simulink model "aero_dap3dof"  (Simulink 6.0)
settings: Solver=ode45  SolverMode=SingleTasking  StartTime=0  StopTime=25  FixedStep=clockt/4  RelTol=1e-3  AbsTol=1e-6
PreLoadFcn:
  | aero_dap3dofdata
values from neighbouring files (symbols this model uses):
  DB = u(6)    [aero_phaseplane.m]
  delt = 0.1    [aero_pointer_tracker.m]
  I = find(diff(Mode.signals.values)~=0)    [aero_guid_plot.m]
undefined symbols (not defined in the file or in its folder): alph1, alphs1, alphsu, alphsv, alphu, alphv, Force, L_arm, tmin
libraries: simulink x2
Description:
  | This model was featured in "Fly Me to the Moon - Then and Now", the story of the digital autopilot in the Lunar Module from the Summer 1999 issue of "MATLAB News & Notes".  You can read the article at:
  | 
  |  http://www.mathworks.com/company/newsletter/news_notes/sum99/lunar_module.html
CloseFcn:
  | h=findobj('type','figure','Name','aero_dap3dof');if ~isempty(h);close(h);end
settings Model: RequirementInfo=9  CovMetricSettings=d  Creator=The MathWorks Inc.  LastModifiedBy=batserve  ExtModeTrigMode=oneshot  ExtModeArmWhenConnect=off  ExtModeAutoUpdateStatusClock=off  ProdHWDeviceType=Specified
settings DataIOCC: LimitDataPoints=off  SignalLoggingName=logsOut
settings OptimizationCC: BlockReduction=off  BooleanDataType=off
settings DebuggingCC: CheckExecutionContextPreStartOutputMsg=on  CheckExecutionContextRuntimeOutputMsg=on  SolverPrmCheckMsg=none
settings HardwareCC: ProdHWDeviceType=Specified
settings RTWCC: TemplateMakefile=grt_vc.tmf

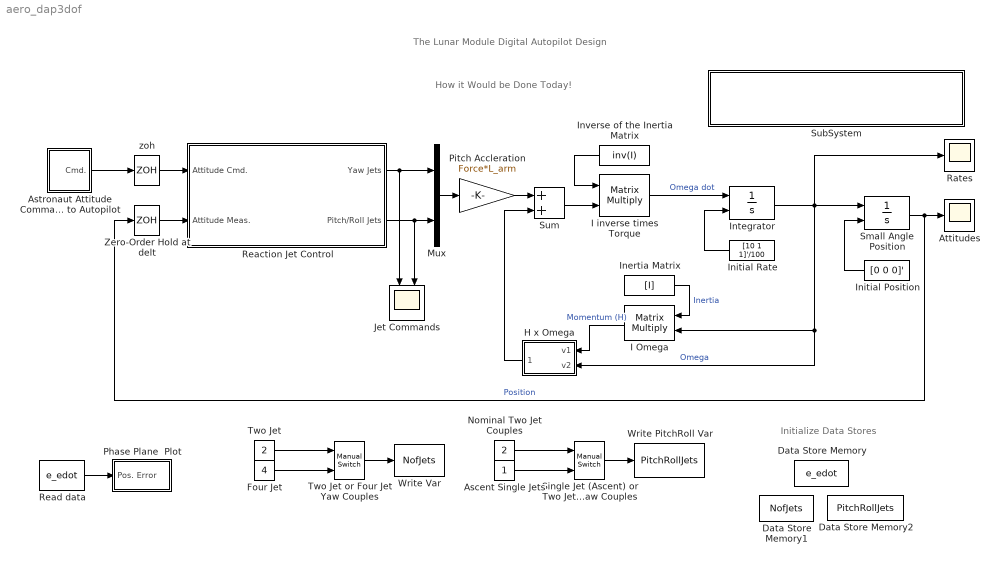
== system aero_dap3dof ==
  note: The Lunar Module Digital Autopilot Design
  note: How it Would be Done Today!
  note: Initialize Data Stores
  Ascent Single Jets : Constant
  Astronaut Attitude Command to Autopilot : Subsystem  PropExecContextAcrossSSBoundary=on
  Attitudes : Scope
      settings: YMin=0  YMax=0.12
  Data Store Memory : DataStoreMemory  DialogController=Simulink.DDGSource  DataStoreName=e_edot  InitialValue=[0 0]
  Data Store Memory1 : DataStoreMemory  DialogController=Simulink.DDGSource  DataStoreName=NofJets  InitialValue=2
  Data Store Memory2 : DataStoreMemory  DialogController=Simulink.DDGSource  DataStoreName=PitchRollJets  InitialValue=2
  Four Jet : Constant  Value=4
  H x Omega : Subsystem  Orientation=left  PropExecContextAcrossSSBoundary=on
      mask Type: Vector Cross Product
      mask Description: This block computes the vector cross product of the first input with the second input.  The output is then z= v1 x v2.
  I Omega : Product  Orientation=left  Multiplication=Matrix(*)  SaturateOnIntegerOverflow=on  RndMeth=Zero  InputSameDT=on
  I inverse times Torque : Product  Multiplication=Matrix(*)  SaturateOnIntegerOverflow=on  RndMeth=Zero  InputSameDT=on
  Inertia Matrix : Constant  Value=[I]  VectorParams1D=off
  Initial Position : Constant  Orientation=left  Value=[0 0 0]'  VectorParams1D=off
  Initial Rate : Constant  Orientation=left  Value=[10 1 1]'/100  VectorParams1D=off
  Integrator : Integrator  InitialConditionSource=external
  Inverse of the Inertia Matrix : Constant  Orientation=left  Value=inv(I)  VectorParams1D=off
  Jet Commands : Scope  NumInputPorts=2
      settings: Orientation=down  TickLabels=on  TimeRange=9.999999999999998  YMin=-3~-3  YMax=3~3  DataFormat=Array  MaxDataPoints=10000
  Mux : Mux  Inputs=2
  Nominal Two Jet Couples : Constant  Value=2
  Phase Plane  Plot : Subsystem  PropExecContextAcrossSSBoundary=on
  Pitch Accleration : Gain  Gain=Force*L_arm  SaturateOnIntegerOverflow=on
  Rates : Scope
      settings: YMin=-0.075  YMax=0.125
  Reaction Jet Control : Subsystem  AncestorBlock=librcs/Reaction Jet Control  PropExecContextAcrossSSBoundary=on
  Read data : DataStoreRead  DialogController=Simulink.DDGSource  DataStoreName=e_edot  SampleTime=delt
  Single Jet (Ascent) or Two Jet Yaw Couples : simulink/Signal Routing/Manual Switch  sw=1  action=0
  Small Angle Position : Integrator  InitialConditionSource=external
  SubSystem : Subsystem  PropExecContextAcrossSSBoundary=on
      mask init:
      | dispstr = sprintf('Read the "News & Notes" article\nabout this model over the web.\n(Double-Click Here)');
      settings: OpenFcn=web http://www.mathworks.com/company/newsletter/news_notes/sum99/lunar_module.html
      mask Display: disp(dispstr)
  Sum : Sum  SaturateOnIntegerOverflow=on  InputSameDT=on
  Two Jet : Constant  Value=2
  Two Jet or Four Jet Yaw Couples : simulink/Signal Routing/Manual Switch  sw=1  action=0
  Write PitchRoll Var : DataStoreWrite  DialogController=Simulink.DDGSource  DataStoreName=PitchRollJets  SampleTime=-1
  Write Var : DataStoreWrite  DialogController=Simulink.DDGSource  DataStoreName=NofJets  SampleTime=-1
  Zero-Order Hold at delt : ZeroOrderHold  SampleTime=delt
  zoh : ZeroOrderHold  SampleTime=delt
  wires:
  Inverse of the Inertia Matrix/1 -> I inverse times Torque/1
  I inverse times Torque/1 -> Integrator/1  "Omega dot"
  Inertia Matrix/1 -> I Omega/1  "Inertia"
  Initial Rate/1 -> Integrator/2
  Initial Position/1 -> Small Angle Position/2
  Integrator/1 -> Small Angle Position/1, I Omega/2, H x Omega/2(v2), Rates/1  "Omega"
  Small Angle Position/1 -> Attitudes/1, Zero-Order Hold at delt/1  "Position"
  Sum/1 -> I inverse times Torque/2
  I Omega/1 -> H x Omega/1(v1)  "Momentum (H)"
  H x Omega/1(v1 x v2) -> Sum/2
  Astronaut Attitude Command to Autopilot/1(Cmd.) -> zoh/1
  Pitch Accleration/1 -> Sum/1
  Mux/1 -> Pitch Accleration/1
  Reaction Jet Control/1(Yaw Jets) -> Mux/1, Jet Commands/1
  Reaction Jet Control/2(Pitch/Roll Jets) -> Mux/2, Jet Commands/2
  zoh/1 -> Reaction Jet Control/1(Attitude Cmd.)
  Zero-Order Hold at delt/1 -> Reaction Jet Control/2(Attitude Meas.)
  Ascent Single Jets/1 -> Single Jet (Ascent) or Two Jet Yaw Couples/2
  Nominal Two Jet Couples/1 -> Single Jet (Ascent) or Two Jet Yaw Couples/1
  Single Jet (Ascent) or Two Jet Yaw Couples/1 -> Write PitchRoll Var/1
  Four Jet/1 -> Two Jet or Four Jet Yaw Couples/2
  Two Jet/1 -> Two Jet or Four Jet Yaw Couples/1
  Two Jet or Four Jet Yaw Couples/1 -> Write Var/1
  Read data/1 -> Phase Plane  Plot/1(Pos. Error)

== system aero_dap3dof/Astronaut Attitude Command to Autopilot ==
  Attitude Cmd at t=0 : Constant  Value=[0 0 0]'  VectorParams1D=off
  Attitude Cmd at t=step : Constant  Value=[0.03 0.05 0.1]'  VectorParams1D=off
  Step : Step  Time=0.25  SampleTime=0
  Switch : Switch  Threshold=0.5  SaturateOnIntegerOverflow=on  InputSameDT=on
  Cmd. : Outport
  wires:
  Step/1 -> Switch/2
  Attitude Cmd at t=step/1 -> Switch/1
  Attitude Cmd at t=0/1 -> Switch/3
  Switch/1 -> Cmd./1

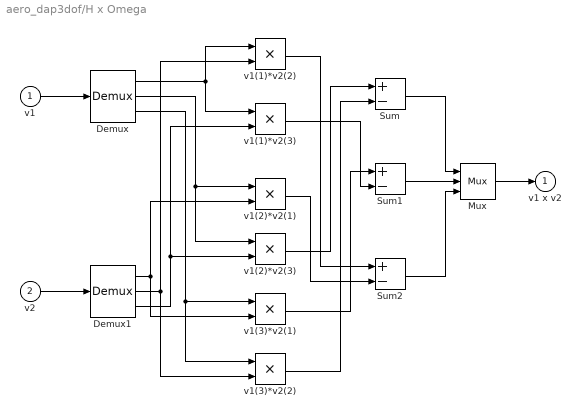
== system aero_dap3dof/H x Omega ==
  v1 : Inport  Port=1  LatchInput=off
  v2 : Inport  Port=2  LatchInput=off
  Demux : Demux  Outputs=3
  Demux1 : Demux  Outputs=3
  Mux : Mux  Inputs=3
  Sum : Sum  Inputs=+-  SaturateOnIntegerOverflow=on  InputSameDT=on
  Sum1 : Sum  Inputs=+-  SaturateOnIntegerOverflow=on  InputSameDT=on
  Sum2 : Sum  Inputs=+-  SaturateOnIntegerOverflow=on  InputSameDT=on
  v1(1)*v2(2) : Product  SaturateOnIntegerOverflow=on  RndMeth=Zero  InputSameDT=on
  v1(1)*v2(3) : Product  SaturateOnIntegerOverflow=on  RndMeth=Zero  InputSameDT=on
  v1(2)*v2(1) : Product  SaturateOnIntegerOverflow=on  RndMeth=Zero  InputSameDT=on
  v1(2)*v2(3) : Product  SaturateOnIntegerOverflow=on  RndMeth=Zero  InputSameDT=on
  v1(3)*v2(1) : Product  SaturateOnIntegerOverflow=on  RndMeth=Zero  InputSameDT=on
  v1(3)*v2(2) : Product  SaturateOnIntegerOverflow=on  RndMeth=Zero  InputSameDT=on
  v1 x v2 : Outport  InitialOutput=0
  wires:
  v1/1 -> Demux/1
  Demux/3 -> v1(3)*v2(1)/1, v1(3)*v2(2)/1
  v2/1 -> Demux1/1
  Demux1/1 -> v1(2)*v2(1)/2, v1(3)*v2(1)/2
  Demux1/2 -> v1(3)*v2(2)/2, v1(1)*v2(2)/2
  Demux1/3 -> v1(2)*v2(3)/2, v1(1)*v2(3)/2
  Demux/1 -> v1(1)*v2(2)/1, v1(1)*v2(3)/1
  Demux/2 -> v1(2)*v2(1)/1, v1(2)*v2(3)/1
  Mux/1 -> v1 x v2/1
  Sum/1 -> Mux/1
  Sum1/1 -> Mux/2
  Sum2/1 -> Mux/3
  v1(2)*v2(3)/1 -> Sum/1
  v1(3)*v2(2)/1 -> Sum/2
  v1(3)*v2(1)/1 -> Sum1/1
  v1(1)*v2(3)/1 -> Sum1/2
  v1(1)*v2(2)/1 -> Sum2/1
  v1(2)*v2(1)/1 -> Sum2/2

== system aero_dap3dof/Phase Plane  Plot ==
  Pos. Error : Inport  Port=1  LatchInput=off
  Constant : Constant  Value=alph1
  Constant1 : Constant  Value=alphs1
  Constants for Plot : Constant  Value=DB
  Digital Clock : DigitalClock  SampleTime=delt
  MATLAB Fcn : MATLABFcn  MATLABFcn=aero_phaseplane  OutputDimensions=0
  Mux1 : Mux  Inputs=5
  wires:
  Mux1/1 -> MATLAB Fcn/1
  Pos. Error/1 -> Mux1/1
  Digital Clock/1 -> Mux1/2
  Constants for Plot/1 -> Mux1/5
  Constant/1 -> Mux1/3
  Constant1/1 -> Mux1/4

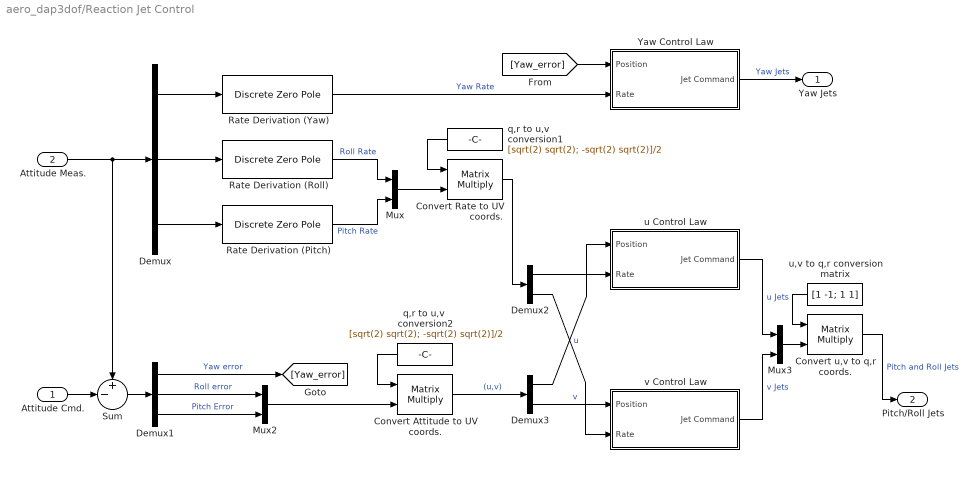
== system aero_dap3dof/Reaction Jet Control ==
  Attitude Cmd. : Inport  Port=1  LatchInput=off
  Attitude Meas. : Inport  Port=2  LatchInput=off
  Convert Attitude to UV coords. : Product  Multiplication=Matrix(*)  SaturateOnIntegerOverflow=on  RndMeth=Zero  InputSameDT=on
  Convert Rate to UV coords. : Product  Multiplication=Matrix(*)  SaturateOnIntegerOverflow=on  RndMeth=Zero  InputSameDT=on
  Convert u,v to q,r coords. : Product  Multiplication=Matrix(*)  SaturateOnIntegerOverflow=on  RndMeth=Zero  InputSameDT=on
  Demux : Demux  Outputs=3
  Demux1 : Demux  Outputs=3
  Demux2 : Demux  Outputs=2
  Demux3 : Demux  Outputs=2
  Mux : Mux  Inputs=2
  Mux2 : Mux  Inputs=2
  Mux3 : Mux  Inputs=2
  Rate Derivation (Pitch) : DiscreteZeroPole  Poles=[0]  Gain=1/delt  SampleTime=-1
  Rate Derivation (Roll) : DiscreteZeroPole  Poles=[0]  Gain=1/delt  SampleTime=-1
  Rate Derivation (Yaw) : DiscreteZeroPole  Poles=[0]  Gain=1/delt  SampleTime=-1
  Sum : Sum  Inputs=+-|  SaturateOnIntegerOverflow=on  InputSameDT=on
  Yaw Control Law : Subsystem  AncestorBlock=libdap/Yaw Control Law  PropExecContextAcrossSSBoundary=on  mask(Control Law){alph=alph1, alphs=alphs1, DB=DB, tmin=tmin, delt=delt}
      mask prompts: alph "Single Jet Accel:"; alphs "Single Jet Switch Curve Accel:"; DB "Dead Band:"; tmin "Min Jet On Time:"; delt "Sample Time:"
      mask help: Implements Control Law for the LM. Works for yaw, u and v jet axes.
  q,r to u,v  conversion1 : Constant  Orientation=left  Value=[sqrt(2) sqrt(2); -sqrt(2) sqrt(2)]/2  VectorParams1D=off
  q,r to u,v  conversion2 : Constant  Orientation=left  Value=[sqrt(2) sqrt(2); -sqrt(2) sqrt(2)]/2  VectorParams1D=off
  u Control Law : Subsystem  AncestorBlock=libdap/Pitch Roll Control Law  PropExecContextAcrossSSBoundary=on  mask(Control Law){alph=alphu, alphs=alphsu, DB=DB, tmin=tmin, delt=delt}
      mask prompts: alph "Single Jet Accel:"; alphs "Single Jet Switch Curve Accel:"; DB "Dead Band:"; tmin "Min. Jet On Time:"; delt "Sample Time:"
      mask help: Implements Control Law for the LM. Works for yaw, u and v jet axes.
  u,v to q,r conversion matrix : Constant  Orientation=left  Value=[1 -1; 1 1]  VectorParams1D=off
  v Control Law : Subsystem  AncestorBlock=libdap/Pitch Roll Control Law  PropExecContextAcrossSSBoundary=on  mask(Control Law){alph=alphv, alphs=alphsv, DB=DB, tmin=tmin, delt=delt}
      mask prompts: alph "Single Jet Accel:"; alphs "Single Jet Switch Curve Accel:"; DB "Dead Band:"; tmin "Min. Jet On Time:"; delt "Sample Time:"
      mask help: Implements Control Law for the LM. Works for yaw, u and v jet axes.
  Yaw Jets : Outport  InitialOutput=0
  Pitch/Roll Jets : Outport  Port=2  InitialOutput=0
  wires:
  q,r to u,v  conversion2/1 -> Convert Attitude to UV coords./1
  q,r to u,v  conversion1/1 -> Convert Rate to UV coords./1
  Rate Derivation (Pitch)/1 -> Mux/2  "Pitch Rate"
  Rate Derivation (Roll)/1 -> Mux/1  "Roll Rate"
  Demux/2 -> Rate Derivation (Roll)/1
  Demux/3 -> Rate Derivation (Pitch)/1
  Demux/1 -> Rate Derivation (Yaw)/1
  Mux/1 -> Convert Rate to UV coords./2
  Attitude Meas./1 -> Demux/1, Sum/1
  Rate Derivation (Yaw)/1 -> Yaw Control Law/2(Rate)  "Yaw Rate"
  Yaw Control Law/1(Jet Command) -> Yaw Jets/1  "Yaw Jets"
  [Yaw_error] -> Yaw Control Law/1(Position)
  Sum/1 -> Demux1/1
  Demux1/2 -> Mux2/1  "Roll error"
  Demux1/3 -> Mux2/2  "Pitch Error"
  Convert Rate to UV coords./1 -> Demux2/1
  Convert Attitude to UV coords./1 -> Demux3/1  "(u,v)"
  Mux2/1 -> Convert Attitude to UV coords./2
  Attitude Cmd./1 -> Sum/2
  v Control Law/1(Jet Command) -> Mux3/2  "v Jets"
  u Control Law/1(Jet Command) -> Mux3/1  "u Jets"
  Demux3/2 -> v Control Law/1(Position)  "v"
  Demux2/1 -> u Control Law/2(Rate)
  Demux1/1 -> [Yaw_error]  "Yaw error"
  Demux2/2 -> v Control Law/2(Rate)
  Mux3/1 -> Convert u,v to q,r coords./2
  u,v to q,r conversion matrix/1 -> Convert u,v to q,r coords./1
  Convert u,v to q,r coords./1 -> Pitch/Roll Jets/1  "Pitch and Roll Jets"
  Demux3/1 -> u Control Law/1(Position)  "u"

== system aero_dap3dof/SubSystem ==

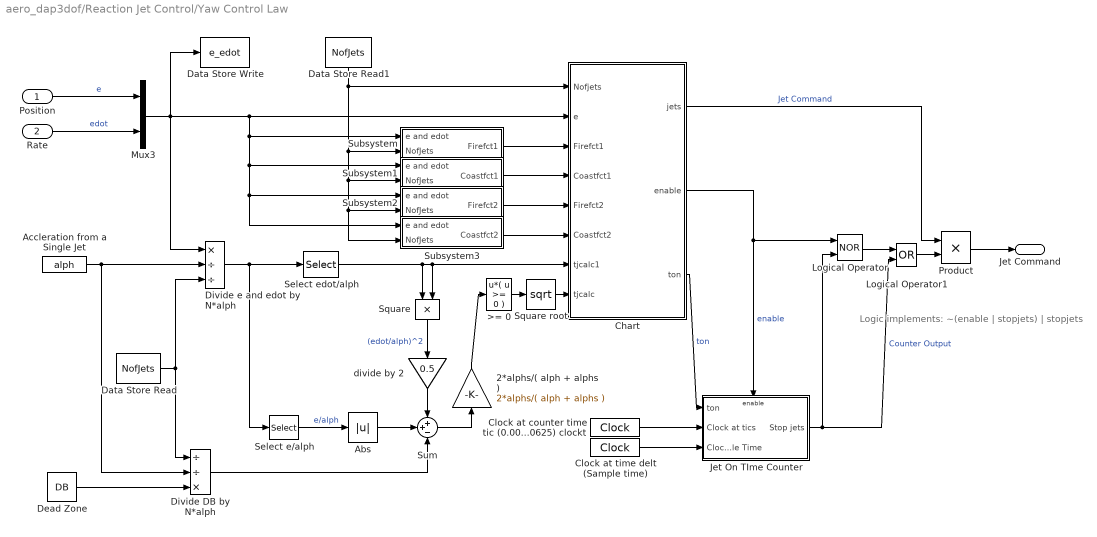
== system aero_dap3dof/Reaction Jet Control/Yaw Control Law ==
  note: Logic implements:
      | ~(enable | stopjets) | stopjets
  Position : Inport  Port=1  LatchInput=off
  Rate : Inport  Port=2  LatchInput=off
  2*alphs/( alph + alphs ) : Gain  Orientation=up  Gain=2*alphs/( alph + alphs )  SaturateOnIntegerOverflow=on
  >= 0 : Fcn  Expr=u*( u >= 0 )
  Abs : Abs  SaturateOnIntegerOverflow=on
  Accleration from a Single Jet : Constant  Value=alph
  Chart : Stateflow chart  PropExecContextAcrossSSBoundary=on
  Clock at counter time tic (0.000625) clockt : DigitalClock  SampleTime=0.000625
  Clock at time delt (Sample time) : DigitalClock  SampleTime=delt
  Data Store Read : DataStoreRead  DialogController=Simulink.DDGSource  DataStoreName=NofJets  SampleTime=delt
  Data Store Read1 : DataStoreRead  Orientation=down  DialogController=Simulink.DDGSource  DataStoreName=NofJets  SampleTime=delt
  Data Store Write : DataStoreWrite  DialogController=Simulink.DDGSource  DataStoreName=e_edot  SampleTime=-1
  Dead Zone : Constant  Value=DB
  Divide e and edot by N*alph : Product  Inputs=*//  SaturateOnIntegerOverflow=on  RndMeth=Zero  InputSameDT=on
  Divide DB by N*alph : Product  Inputs=//*  SaturateOnIntegerOverflow=on  RndMeth=Zero  InputSameDT=on
  Jet On TIme Counter : Subsystem  TreatAsAtomicUnit=on  PropExecContextAcrossSSBoundary=on
  Logical Operator : Logic  Operator=NOR
  Logical Operator1 : Logic  Operator=OR
  Mux3 : Mux  Inputs=2
  Product : Product  SaturateOnIntegerOverflow=on  RndMeth=Zero  InputSameDT=on
  Select e/alph : Selector  Elements=[1]  InputPortWidth=2
  Select edot/alph : Selector  Elements=[2]  InputPortWidth=2
  Square : Product  Orientation=down  SaturateOnIntegerOverflow=on  RndMeth=Zero  InputSameDT=on
  Square root : Math  Operator=sqrt  SaturateOnIntegerOverflow=on
  Subsystem : Subsystem  PropExecContextAcrossSSBoundary=on
  Subsystem1 : Subsystem  PropExecContextAcrossSSBoundary=on
  Subsystem2 : Subsystem  PropExecContextAcrossSSBoundary=on
  Subsystem3 : Subsystem  PropExecContextAcrossSSBoundary=on
  Sum : Sum  Inputs=++-  SaturateOnIntegerOverflow=on  InputSameDT=on
  divide by 2 : Gain  Orientation=down  Gain=0.5  SaturateOnIntegerOverflow=on
  Jet Command : Outport  InitialOutput=0
  wires:
  >= 0/1 -> Square root/1
  2*alphs/( alph + alphs )/1 -> >= 0/1
  Data Store Read1/1 -> Subsystem3/2(NofJets), Subsystem2/2(NofJets), Subsystem1/2(NofJets), Subsystem/2(NofJets), Chart/1(Nofjets)
  Rate/1 -> Mux3/2  "edot"
  Position/1 -> Mux3/1  "e"
  Mux3/1 -> Data Store Write/1, Chart/2(e), Divide e and edot by N*alph/1, Subsystem/1(e and edot), Subsystem1/1(e and edot), Subsystem2/1(e and edot), Subsystem3/1(e and edot)
  Square/1 -> divide by 2/1  "(edot/alph)^2"
  Square root/1 -> Chart/8(tjcalc)
  Chart/1(jets) -> Product/1  "Jet Command"
  Select edot/alph/1 -> Square/1, Chart/7(tjcalc1), Square/2
  Select e/alph/1 -> Abs/1  "e/alph"
  divide by 2/1 -> Sum/1
  Sum/1 -> 2*alphs/( alph + alphs )/1
  Abs/1 -> Sum/2
  Divide e and edot by N*alph/1 -> Select edot/alph/1, Select e/alph/1
  Data Store Read/1 -> Divide e and edot by N*alph/3, Divide DB by N*alph/1
  Accleration from a Single Jet/1 -> Divide e and edot by N*alph/2, Divide DB by N*alph/2
  Dead Zone/1 -> Divide DB by N*alph/3
  Divide DB by N*alph/1 -> Sum/3
  Chart/2(enable) -> Jet On TIme Counter/Enable, Logical Operator/1  "enable"
  Logical Operator1/1 -> Product/2
  Chart/3(ton) -> Jet On TIme Counter/1(ton)  "ton"
  Clock at counter time tic (0.000625) clockt/1 -> Jet On TIme Counter/2(Clock at tics)
  Clock at time delt (Sample time)/1 -> Jet On TIme Counter/3(Clock at Sample Time)
  Jet On TIme Counter/1(Stop jets) -> Logical Operator/2, Logical Operator1/2  "Counter Output"
  Logical Operator/1 -> Logical Operator1/1
  Subsystem3/1(Coastfct2) -> Chart/6(Coastfct2)
  Subsystem2/1(Firefct2) -> Chart/5(Firefct2)
  Subsystem1/1(Coastfct1) -> Chart/4(Coastfct1)
  Subsystem/1(Firefct1) -> Chart/3(Firefct1)
  Product/1 -> Jet Command/1

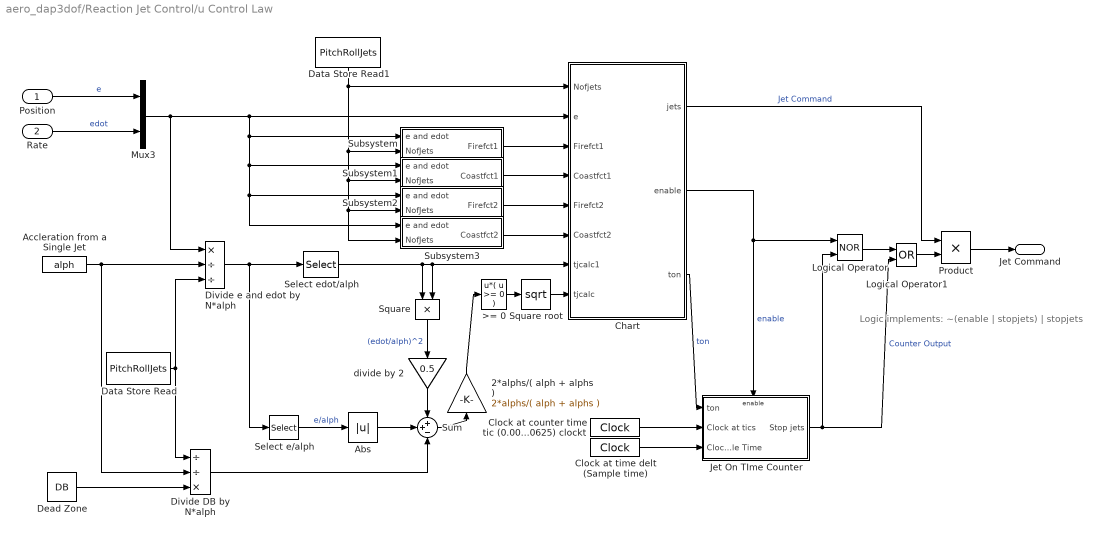
== system aero_dap3dof/Reaction Jet Control/u Control Law ==
  note: Logic implements:
      | ~(enable | stopjets) | stopjets
  Position : Inport  Port=1  LatchInput=off
  Rate : Inport  Port=2  LatchInput=off
  2*alphs/( alph + alphs ) : Gain  Orientation=up  Gain=2*alphs/( alph + alphs )  SaturateOnIntegerOverflow=on
  >= 0 : Fcn  Expr=u*( u >= 0 )
  Abs : Abs  SaturateOnIntegerOverflow=on
  Accleration from a Single Jet : Constant  Value=alph
  Chart : Stateflow chart  PropExecContextAcrossSSBoundary=on
  Clock at counter time tic (0.000625) clockt : DigitalClock  SampleTime=0.000625
  Clock at time delt (Sample time) : DigitalClock  SampleTime=delt
  Data Store Read : DataStoreRead  DialogController=Simulink.DDGSource  DataStoreName=PitchRollJets  SampleTime=delt
  Data Store Read1 : DataStoreRead  Orientation=down  DialogController=Simulink.DDGSource  DataStoreName=PitchRollJets  SampleTime=delt
  Dead Zone : Constant  Value=DB
  Divide e and edot by N*alph : Product  Inputs=*//  SaturateOnIntegerOverflow=on  RndMeth=Zero  InputSameDT=on
  Divide DB by N*alph : Product  Inputs=//*  SaturateOnIntegerOverflow=on  RndMeth=Zero  InputSameDT=on
  Jet On TIme Counter : Subsystem  TreatAsAtomicUnit=on  PropExecContextAcrossSSBoundary=on
  Logical Operator : Logic  Operator=NOR
  Logical Operator1 : Logic  Operator=OR
  Mux3 : Mux  Inputs=2
  Product : Product  SaturateOnIntegerOverflow=on  RndMeth=Zero  InputSameDT=on
  Select e/alph : Selector  Elements=[1]  InputPortWidth=2
  Select edot/alph : Selector  Elements=[2]  InputPortWidth=2
  Square : Product  Orientation=down  SaturateOnIntegerOverflow=on  RndMeth=Zero  InputSameDT=on
  Square root : Math  Operator=sqrt  SaturateOnIntegerOverflow=on
  Subsystem : Subsystem  PropExecContextAcrossSSBoundary=on
  Subsystem1 : Subsystem  PropExecContextAcrossSSBoundary=on
  Subsystem2 : Subsystem  PropExecContextAcrossSSBoundary=on
  Subsystem3 : Subsystem  PropExecContextAcrossSSBoundary=on
  Sum : Sum  Inputs=++-  SaturateOnIntegerOverflow=on  InputSameDT=on
  divide by 2 : Gain  Orientation=down  Gain=0.5  SaturateOnIntegerOverflow=on
  Jet Command : Outport  InitialOutput=0
  wires:
  >= 0/1 -> Square root/1
  2*alphs/( alph + alphs )/1 -> >= 0/1
  Product/1 -> Jet Command/1
  Subsystem/1(Firefct1) -> Chart/3(Firefct1)
  Subsystem1/1(Coastfct1) -> Chart/4(Coastfct1)
  Subsystem2/1(Firefct2) -> Chart/5(Firefct2)
  Subsystem3/1(Coastfct2) -> Chart/6(Coastfct2)
  Logical Operator/1 -> Logical Operator1/1
  Jet On TIme Counter/1(Stop jets) -> Logical Operator1/2, Logical Operator/2  "Counter Output"
  Clock at time delt (Sample time)/1 -> Jet On TIme Counter/3(Clock at Sample Time)
  Clock at counter time tic (0.000625) clockt/1 -> Jet On TIme Counter/2(Clock at tics)
  Chart/3(ton) -> Jet On TIme Counter/1(ton)  "ton"
  Logical Operator1/1 -> Product/2
  Chart/2(enable) -> Logical Operator/1, Jet On TIme Counter/Enable  "enable"
  Divide DB by N*alph/1 -> Sum/3
  Dead Zone/1 -> Divide DB by N*alph/3
  Accleration from a Single Jet/1 -> Divide DB by N*alph/2, Divide e and edot by N*alph/2
  Data Store Read/1 -> Divide DB by N*alph/1, Divide e and edot by N*alph/3
  Divide e and edot by N*alph/1 -> Select e/alph/1, Select edot/alph/1
  Abs/1 -> Sum/2
  Sum/1 -> 2*alphs/( alph + alphs )/1
  divide by 2/1 -> Sum/1
  Select e/alph/1 -> Abs/1  "e/alph"
  Select edot/alph/1 -> Square/2, Chart/7(tjcalc1), Square/1
  Chart/1(jets) -> Product/1  "Jet Command"
  Square root/1 -> Chart/8(tjcalc)
  Square/1 -> divide by 2/1  "(edot/alph)^2"
  Mux3/1 -> Subsystem3/1(e and edot), Subsystem2/1(e and edot), Subsystem1/1(e and edot), Subsystem/1(e and edot), Divide e and edot by N*alph/1, Chart/2(e)
  Position/1 -> Mux3/1  "e"
  Rate/1 -> Mux3/2  "edot"
  Data Store Read1/1 -> Chart/1(Nofjets), Subsystem/2(NofJets), Subsystem1/2(NofJets), Subsystem2/2(NofJets), Subsystem3/2(NofJets)

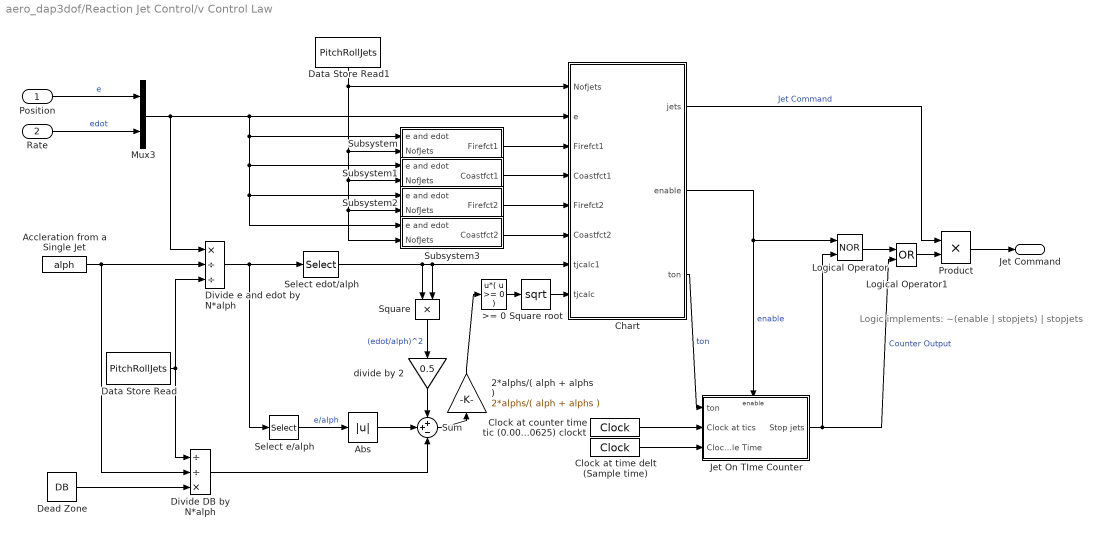
== system aero_dap3dof/Reaction Jet Control/v Control Law ==
  note: Logic implements:
      | ~(enable | stopjets) | stopjets
  Position : Inport  Port=1  LatchInput=off
  Rate : Inport  Port=2  LatchInput=off
  2*alphs/( alph + alphs ) : Gain  Orientation=up  Gain=2*alphs/( alph + alphs )  SaturateOnIntegerOverflow=on
  >= 0 : Fcn  Expr=u*( u >= 0 )
  Abs : Abs  SaturateOnIntegerOverflow=on
  Accleration from a Single Jet : Constant  Value=alph
  Chart : Stateflow chart  PropExecContextAcrossSSBoundary=on
  Clock at counter time tic (0.000625) clockt : DigitalClock  SampleTime=0.000625
  Clock at time delt (Sample time) : DigitalClock  SampleTime=delt
  Data Store Read : DataStoreRead  DialogController=Simulink.DDGSource  DataStoreName=PitchRollJets  SampleTime=delt
  Data Store Read1 : DataStoreRead  Orientation=down  DialogController=Simulink.DDGSource  DataStoreName=PitchRollJets  SampleTime=delt
  Dead Zone : Constant  Value=DB
  Divide e and edot by N*alph : Product  Inputs=*//  SaturateOnIntegerOverflow=on  RndMeth=Zero  InputSameDT=on
  Divide DB by N*alph : Product  Inputs=//*  SaturateOnIntegerOverflow=on  RndMeth=Zero  InputSameDT=on
  Jet On TIme Counter : Subsystem  TreatAsAtomicUnit=on  PropExecContextAcrossSSBoundary=on
  Logical Operator : Logic  Operator=NOR
  Logical Operator1 : Logic  Operator=OR
  Mux3 : Mux  Inputs=2
  Product : Product  SaturateOnIntegerOverflow=on  RndMeth=Zero  InputSameDT=on
  Select e/alph : Selector  Elements=[1]  InputPortWidth=2
  Select edot/alph : Selector  Elements=[2]  InputPortWidth=2
  Square : Product  Orientation=down  SaturateOnIntegerOverflow=on  RndMeth=Zero  InputSameDT=on
  Square root : Math  Operator=sqrt  SaturateOnIntegerOverflow=on
  Subsystem : Subsystem  PropExecContextAcrossSSBoundary=on
  Subsystem1 : Subsystem  PropExecContextAcrossSSBoundary=on
  Subsystem2 : Subsystem  PropExecContextAcrossSSBoundary=on
  Subsystem3 : Subsystem  PropExecContextAcrossSSBoundary=on
  Sum : Sum  Inputs=++-  SaturateOnIntegerOverflow=on  InputSameDT=on
  divide by 2 : Gain  Orientation=down  Gain=0.5  SaturateOnIntegerOverflow=on
  Jet Command : Outport  InitialOutput=0
  wires:
  >= 0/1 -> Square root/1
  2*alphs/( alph + alphs )/1 -> >= 0/1
  Product/1 -> Jet Command/1
  Subsystem/1(Firefct1) -> Chart/3(Firefct1)
  Subsystem1/1(Coastfct1) -> Chart/4(Coastfct1)
  Subsystem2/1(Firefct2) -> Chart/5(Firefct2)
  Subsystem3/1(Coastfct2) -> Chart/6(Coastfct2)
  Logical Operator/1 -> Logical Operator1/1
  Jet On TIme Counter/1(Stop jets) -> Logical Operator1/2, Logical Operator/2  "Counter Output"
  Clock at time delt (Sample time)/1 -> Jet On TIme Counter/3(Clock at Sample Time)
  Clock at counter time tic (0.000625) clockt/1 -> Jet On TIme Counter/2(Clock at tics)
  Chart/3(ton) -> Jet On TIme Counter/1(ton)  "ton"
  Logical Operator1/1 -> Product/2
  Chart/2(enable) -> Logical Operator/1, Jet On TIme Counter/Enable  "enable"
  Divide DB by N*alph/1 -> Sum/3
  Dead Zone/1 -> Divide DB by N*alph/3
  Accleration from a Single Jet/1 -> Divide DB by N*alph/2, Divide e and edot by N*alph/2
  Data Store Read/1 -> Divide DB by N*alph/1, Divide e and edot by N*alph/3
  Divide e and edot by N*alph/1 -> Select e/alph/1, Select edot/alph/1
  Abs/1 -> Sum/2
  Sum/1 -> 2*alphs/( alph + alphs )/1
  divide by 2/1 -> Sum/1
  Select e/alph/1 -> Abs/1  "e/alph"
  Select edot/alph/1 -> Square/2, Chart/7(tjcalc1), Square/1
  Chart/1(jets) -> Product/1  "Jet Command"
  Square root/1 -> Chart/8(tjcalc)
  Square/1 -> divide by 2/1  "(edot/alph)^2"
  Mux3/1 -> Subsystem3/1(e and edot), Subsystem2/1(e and edot), Subsystem1/1(e and edot), Subsystem/1(e and edot), Divide e and edot by N*alph/1, Chart/2(e)
  Position/1 -> Mux3/1  "e"
  Rate/1 -> Mux3/2  "edot"
  Data Store Read1/1 -> Chart/1(Nofjets), Subsystem/2(NofJets), Subsystem1/2(NofJets), Subsystem2/2(NofJets), Subsystem3/2(NofJets)

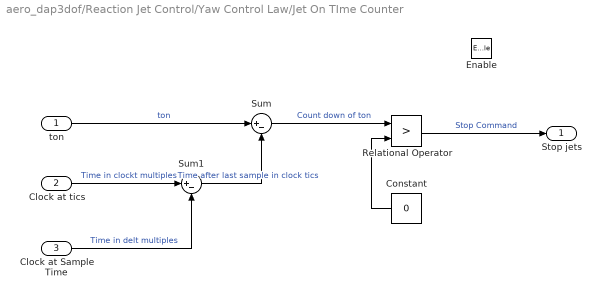
== system aero_dap3dof/Reaction Jet Control/Yaw Control Law/Jet On TIme Counter ==
  ton : Inport  Port=1  LatchInput=off
  Clock at tics : Inport  Port=2  LatchInput=off
  Clock at Sample Time : Inport  Port=3  LatchInput=off
  Enable : EnablePort  StatesWhenEnabling=reset
  Constant : Constant  Orientation=left  Value=0
  Relational Operator : RelationalOperator  Operator=>  InputSameDT=on
  Sum : Sum  Inputs=|+-  SaturateOnIntegerOverflow=on  InputSameDT=on
  Sum1 : Sum  Inputs=|+-  SaturateOnIntegerOverflow=on  InputSameDT=on
  Stop jets : Outport
  wires:
  Constant/1 -> Relational Operator/2
  ton/1 -> Sum/1  "ton"
  Clock at tics/1 -> Sum1/1  "Time in clockt multiples"
  Clock at Sample Time/1 -> Sum1/2  "Time in delt multiples"
  Sum1/1 -> Sum/2  "Time after last sample in clock tics"
  Sum/1 -> Relational Operator/1  "Count down of ton"
  Relational Operator/1 -> Stop jets/1  "Stop Command"

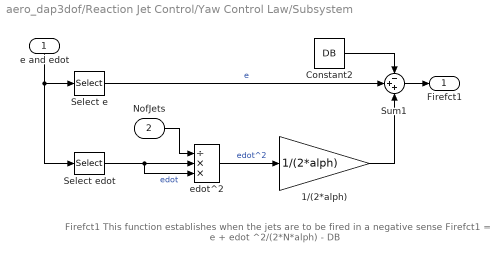
== system aero_dap3dof/Reaction Jet Control/Yaw Control Law/Subsystem ==
  note: Firefct1
      | This function establishes when the jets are to be fired in a negative sense
      | Firefct1 = e + edot ^2/(2*N*alph) - DB
  e and edot : Inport  Orientation=down  Port=1  LatchInput=off
  NofJets : Inport  Port=2  LatchInput=off
  1/(2*alph) : Gain  Gain=1/(2*alph)  SaturateOnIntegerOverflow=on
  Constant2 : Constant  Value=DB
  Select e : Selector  Elements=[1]  InputPortWidth=2
  Select edot : Selector  Elements=[2]  InputPortWidth=2
  Sum1 : Sum  Inputs=-++  SaturateOnIntegerOverflow=on  InputSameDT=on
  edot^2 : Product  Inputs=/**  SaturateOnIntegerOverflow=on  RndMeth=Zero  InputSameDT=on
  Firefct1 : Outport
  wires:
  edot^2/1 -> 1/(2*alph)/1  "edot^2"
  Select edot/1 -> edot^2/2, edot^2/3  "edot"
  NofJets/1 -> edot^2/1
  e and edot/1 -> Select e/1, Select edot/1
  1/(2*alph)/1 -> Sum1/3
  Constant2/1 -> Sum1/1
  Select e/1 -> Sum1/2  "e"
  Sum1/1 -> Firefct1/1

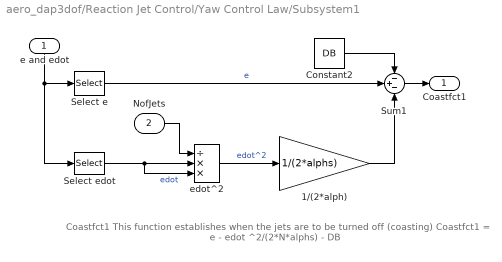
== system aero_dap3dof/Reaction Jet Control/Yaw Control Law/Subsystem1 ==
  note: Coastfct1
      | This function establishes when the jets are to be turned off (coasting)
      | Coastfct1 = e - edot ^2/(2*N*alphs) - DB
  e and edot : Inport  Orientation=down  Port=1  LatchInput=off
  NofJets : Inport  Port=2  LatchInput=off
  1/(2*alph) : Gain  Gain=1/(2*alphs)  SaturateOnIntegerOverflow=on
  Constant2 : Constant  Value=DB
  Select e : Selector  Elements=[1]  InputPortWidth=2
  Select edot : Selector  Elements=[2]  InputPortWidth=2
  Sum1 : Sum  Inputs=-+-  SaturateOnIntegerOverflow=on  InputSameDT=on
  edot^2 : Product  Inputs=/**  SaturateOnIntegerOverflow=on  RndMeth=Zero  InputSameDT=on
  Coastfct1 : Outport
  wires:
  Sum1/1 -> Coastfct1/1
  Select e/1 -> Sum1/2  "e"
  Constant2/1 -> Sum1/1
  1/(2*alph)/1 -> Sum1/3
  e and edot/1 -> Select edot/1, Select e/1
  NofJets/1 -> edot^2/1
  Select edot/1 -> edot^2/3, edot^2/2  "edot"
  edot^2/1 -> 1/(2*alph)/1  "edot^2"

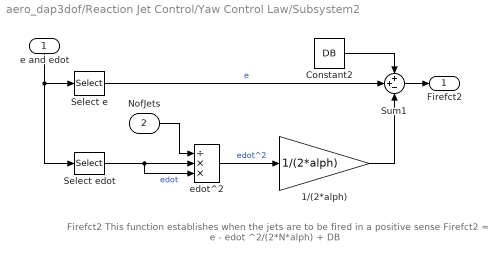
== system aero_dap3dof/Reaction Jet Control/Yaw Control Law/Subsystem2 ==
  note: Firefct2
      | This function establishes when the jets are to be fired in a positive sense
      | Firefct2 = e - edot ^2/(2*N*alph) + DB
  e and edot : Inport  Orientation=down  Port=1  LatchInput=off
  NofJets : Inport  Port=2  LatchInput=off
  1/(2*alph) : Gain  Gain=1/(2*alph)  SaturateOnIntegerOverflow=on
  Constant2 : Constant  Value=DB
  Select e : Selector  Elements=[1]  InputPortWidth=2
  Select edot : Selector  Elements=[2]  InputPortWidth=2
  Sum1 : Sum  Inputs=++-  SaturateOnIntegerOverflow=on  InputSameDT=on
  edot^2 : Product  Inputs=/**  SaturateOnIntegerOverflow=on  RndMeth=Zero  InputSameDT=on
  Firefct2 : Outport
  wires:
  edot^2/1 -> 1/(2*alph)/1  "edot^2"
  Select edot/1 -> edot^2/2, edot^2/3  "edot"
  NofJets/1 -> edot^2/1
  e and edot/1 -> Select e/1, Select edot/1
  1/(2*alph)/1 -> Sum1/3
  Constant2/1 -> Sum1/1
  Select e/1 -> Sum1/2  "e"
  Sum1/1 -> Firefct2/1

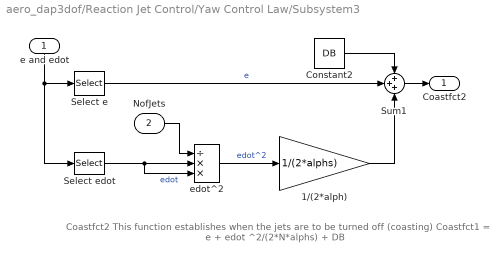
== system aero_dap3dof/Reaction Jet Control/Yaw Control Law/Subsystem3 ==
  note: Coastfct2
      | This function establishes when the jets are to be turned off (coasting)
      | Coastfct1 = e + edot ^2/(2*N*alphs) + DB
  e and edot : Inport  Orientation=down  Port=1  LatchInput=off
  NofJets : Inport  Port=2  LatchInput=off
  1/(2*alph) : Gain  Gain=1/(2*alphs)  SaturateOnIntegerOverflow=on
  Constant2 : Constant  Value=DB
  Select e : Selector  Elements=[1]  InputPortWidth=2
  Select edot : Selector  Elements=[2]  InputPortWidth=2
  Sum1 : Sum  Inputs=+++  SaturateOnIntegerOverflow=on  InputSameDT=on
  edot^2 : Product  Inputs=/**  SaturateOnIntegerOverflow=on  RndMeth=Zero  InputSameDT=on
  Coastfct2 : Outport
  wires:
  edot^2/1 -> 1/(2*alph)/1  "edot^2"
  Select edot/1 -> edot^2/2, edot^2/3  "edot"
  NofJets/1 -> edot^2/1
  e and edot/1 -> Select e/1, Select edot/1
  1/(2*alph)/1 -> Sum1/3
  Constant2/1 -> Sum1/1
  Select e/1 -> Sum1/2  "e"
  Sum1/1 -> Coastfct2/1

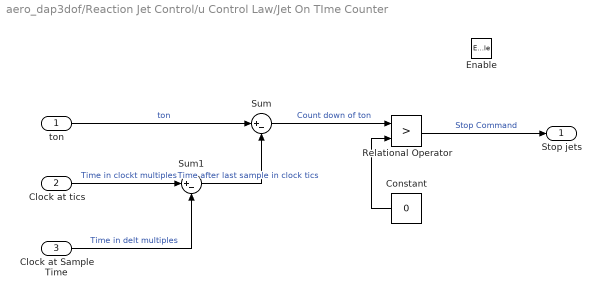
== system aero_dap3dof/Reaction Jet Control/u Control Law/Jet On TIme Counter ==
  ton : Inport  Port=1  LatchInput=off
  Clock at tics : Inport  Port=2  LatchInput=off
  Clock at Sample Time : Inport  Port=3  LatchInput=off
  Enable : EnablePort  StatesWhenEnabling=reset
  Constant : Constant  Orientation=left  Value=0
  Relational Operator : RelationalOperator  Operator=>  InputSameDT=on
  Sum : Sum  Inputs=|+-  SaturateOnIntegerOverflow=on  InputSameDT=on
  Sum1 : Sum  Inputs=|+-  SaturateOnIntegerOverflow=on  InputSameDT=on
  Stop jets : Outport
  wires:
  Relational Operator/1 -> Stop jets/1  "Stop Command"
  Sum/1 -> Relational Operator/1  "Count down of ton"
  Sum1/1 -> Sum/2  "Time after last sample in clock tics"
  Clock at Sample Time/1 -> Sum1/2  "Time in delt multiples"
  Clock at tics/1 -> Sum1/1  "Time in clockt multiples"
  ton/1 -> Sum/1  "ton"
  Constant/1 -> Relational Operator/2

== system aero_dap3dof/Reaction Jet Control/u Control Law/Subsystem ==
  note: Firefct1
      | This function establishes when the jets are to be fired in a negative sense
      | Firefct1 = e + edot ^2/(2*N*alph) - DB
  e and edot : Inport  Orientation=down  Port=1  LatchInput=off
  NofJets : Inport  Port=2  LatchInput=off
  1/(2*alph) : Gain  Gain=1/(2*alph)  SaturateOnIntegerOverflow=on
  Constant2 : Constant  Value=DB
  Select e : Selector  Elements=[1]  InputPortWidth=2
  Select edot : Selector  Elements=[2]  InputPortWidth=2
  Sum1 : Sum  Inputs=-++  SaturateOnIntegerOverflow=on  InputSameDT=on
  edot^2 : Product  Inputs=/**  SaturateOnIntegerOverflow=on  RndMeth=Zero  InputSameDT=on
  Firefct1 : Outport
  wires:
  Sum1/1 -> Firefct1/1
  Select e/1 -> Sum1/2  "e"
  Constant2/1 -> Sum1/1
  1/(2*alph)/1 -> Sum1/3
  e and edot/1 -> Select edot/1, Select e/1
  NofJets/1 -> edot^2/1
  Select edot/1 -> edot^2/3, edot^2/2  "edot"
  edot^2/1 -> 1/(2*alph)/1  "edot^2"

== system aero_dap3dof/Reaction Jet Control/u Control Law/Subsystem1 ==
  note: Coastfct1
      | This function establishes when the jets are to be turned off (coasting)
      | Coastfct1 = e - edot ^2/(2*N*alphs) - DB
  e and edot : Inport  Orientation=down  Port=1  LatchInput=off
  NofJets : Inport  Port=2  LatchInput=off
  1/(2*alph) : Gain  Gain=1/(2*alphs)  SaturateOnIntegerOverflow=on
  Constant2 : Constant  Value=DB
  Select e : Selector  Elements=[1]  InputPortWidth=2
  Select edot : Selector  Elements=[2]  InputPortWidth=2
  Sum1 : Sum  Inputs=-+-  SaturateOnIntegerOverflow=on  InputSameDT=on
  edot^2 : Product  Inputs=/**  SaturateOnIntegerOverflow=on  RndMeth=Zero  InputSameDT=on
  Coastfct1 : Outport
  wires:
  edot^2/1 -> 1/(2*alph)/1  "edot^2"
  Select edot/1 -> edot^2/2, edot^2/3  "edot"
  NofJets/1 -> edot^2/1
  e and edot/1 -> Select e/1, Select edot/1
  1/(2*alph)/1 -> Sum1/3
  Constant2/1 -> Sum1/1
  Select e/1 -> Sum1/2  "e"
  Sum1/1 -> Coastfct1/1

== system aero_dap3dof/Reaction Jet Control/u Control Law/Subsystem2 ==
  note: Firefct2
      | This function establishes when the jets are to be fired in a positive sense
      | Firefct2 = e - edot ^2/(2*N*alph) + DB
  e and edot : Inport  Orientation=down  Port=1  LatchInput=off
  NofJets : Inport  Port=2  LatchInput=off
  1/(2*alph) : Gain  Gain=1/(2*alph)  SaturateOnIntegerOverflow=on
  Constant2 : Constant  Value=DB
  Select e : Selector  Elements=[1]  InputPortWidth=2
  Select edot : Selector  Elements=[2]  InputPortWidth=2
  Sum1 : Sum  Inputs=++-  SaturateOnIntegerOverflow=on  InputSameDT=on
  edot^2 : Product  Inputs=/**  SaturateOnIntegerOverflow=on  RndMeth=Zero  InputSameDT=on
  Firefct2 : Outport
  wires:
  Sum1/1 -> Firefct2/1
  Select e/1 -> Sum1/2  "e"
  Constant2/1 -> Sum1/1
  1/(2*alph)/1 -> Sum1/3
  e and edot/1 -> Select edot/1, Select e/1
  NofJets/1 -> edot^2/1
  Select edot/1 -> edot^2/3, edot^2/2  "edot"
  edot^2/1 -> 1/(2*alph)/1  "edot^2"

== system aero_dap3dof/Reaction Jet Control/u Control Law/Subsystem3 ==
  note: Coastfct2
      | This function establishes when the jets are to be turned off (coasting)
      | Coastfct1 = e + edot ^2/(2*N*alphs) + DB
  e and edot : Inport  Orientation=down  Port=1  LatchInput=off
  NofJets : Inport  Port=2  LatchInput=off
  1/(2*alph) : Gain  Gain=1/(2*alphs)  SaturateOnIntegerOverflow=on
  Constant2 : Constant  Value=DB
  Select e : Selector  Elements=[1]  InputPortWidth=2
  Select edot : Selector  Elements=[2]  InputPortWidth=2
  Sum1 : Sum  Inputs=+++  SaturateOnIntegerOverflow=on  InputSameDT=on
  edot^2 : Product  Inputs=/**  SaturateOnIntegerOverflow=on  RndMeth=Zero  InputSameDT=on
  Coastfct2 : Outport
  wires:
  Sum1/1 -> Coastfct2/1
  Select e/1 -> Sum1/2  "e"
  Constant2/1 -> Sum1/1
  1/(2*alph)/1 -> Sum1/3
  e and edot/1 -> Select edot/1, Select e/1
  NofJets/1 -> edot^2/1
  Select edot/1 -> edot^2/3, edot^2/2  "edot"
  edot^2/1 -> 1/(2*alph)/1  "edot^2"

== system aero_dap3dof/Reaction Jet Control/v Control Law/Jet On TIme Counter ==
  ton : Inport  Port=1  LatchInput=off
  Clock at tics : Inport  Port=2  LatchInput=off
  Clock at Sample Time : Inport  Port=3  LatchInput=off
  Enable : EnablePort  StatesWhenEnabling=reset
  Constant : Constant  Orientation=left  Value=0
  Relational Operator : RelationalOperator  Operator=>  InputSameDT=on
  Sum : Sum  Inputs=|+-  SaturateOnIntegerOverflow=on  InputSameDT=on
  Sum1 : Sum  Inputs=|+-  SaturateOnIntegerOverflow=on  InputSameDT=on
  Stop jets : Outport
  wires:
  Relational Operator/1 -> Stop jets/1  "Stop Command"
  Sum/1 -> Relational Operator/1  "Count down of ton"
  Sum1/1 -> Sum/2  "Time after last sample in clock tics"
  Clock at Sample Time/1 -> Sum1/2  "Time in delt multiples"
  Clock at tics/1 -> Sum1/1  "Time in clockt multiples"
  ton/1 -> Sum/1  "ton"
  Constant/1 -> Relational Operator/2

== system aero_dap3dof/Reaction Jet Control/v Control Law/Subsystem ==
  note: Firefct1
      | This function establishes when the jets are to be fired in a negative sense
      | Firefct1 = e + edot ^2/(2*N*alph) - DB
  e and edot : Inport  Orientation=down  Port=1  LatchInput=off
  NofJets : Inport  Port=2  LatchInput=off
  1/(2*alph) : Gain  Gain=1/(2*alph)  SaturateOnIntegerOverflow=on
  Constant2 : Constant  Value=DB
  Select e : Selector  Elements=[1]  InputPortWidth=2
  Select edot : Selector  Elements=[2]  InputPortWidth=2
  Sum1 : Sum  Inputs=-++  SaturateOnIntegerOverflow=on  InputSameDT=on
  edot^2 : Product  Inputs=/**  SaturateOnIntegerOverflow=on  RndMeth=Zero  InputSameDT=on
  Firefct1 : Outport
  wires:
  Sum1/1 -> Firefct1/1
  Select e/1 -> Sum1/2  "e"
  Constant2/1 -> Sum1/1
  1/(2*alph)/1 -> Sum1/3
  e and edot/1 -> Select edot/1, Select e/1
  NofJets/1 -> edot^2/1
  Select edot/1 -> edot^2/3, edot^2/2  "edot"
  edot^2/1 -> 1/(2*alph)/1  "edot^2"

== system aero_dap3dof/Reaction Jet Control/v Control Law/Subsystem1 ==
  note: Coastfct1
      | This function establishes when the jets are to be turned off (coasting)
      | Coastfct1 = e - edot ^2/(2*N*alphs) - DB
  e and edot : Inport  Orientation=down  Port=1  LatchInput=off
  NofJets : Inport  Port=2  LatchInput=off
  1/(2*alph) : Gain  Gain=1/(2*alphs)  SaturateOnIntegerOverflow=on
  Constant2 : Constant  Value=DB
  Select e : Selector  Elements=[1]  InputPortWidth=2
  Select edot : Selector  Elements=[2]  InputPortWidth=2
  Sum1 : Sum  Inputs=-+-  SaturateOnIntegerOverflow=on  InputSameDT=on
  edot^2 : Product  Inputs=/**  SaturateOnIntegerOverflow=on  RndMeth=Zero  InputSameDT=on
  Coastfct1 : Outport
  wires:
  edot^2/1 -> 1/(2*alph)/1  "edot^2"
  Select edot/1 -> edot^2/2, edot^2/3  "edot"
  NofJets/1 -> edot^2/1
  e and edot/1 -> Select e/1, Select edot/1
  1/(2*alph)/1 -> Sum1/3
  Constant2/1 -> Sum1/1
  Select e/1 -> Sum1/2  "e"
  Sum1/1 -> Coastfct1/1

== system aero_dap3dof/Reaction Jet Control/v Control Law/Subsystem2 ==
  note: Firefct2
      | This function establishes when the jets are to be fired in a positive sense
      | Firefct2 = e - edot ^2/(2*N*alph) + DB
  e and edot : Inport  Orientation=down  Port=1  LatchInput=off
  NofJets : Inport  Port=2  LatchInput=off
  1/(2*alph) : Gain  Gain=1/(2*alph)  SaturateOnIntegerOverflow=on
  Constant2 : Constant  Value=DB
  Select e : Selector  Elements=[1]  InputPortWidth=2
  Select edot : Selector  Elements=[2]  InputPortWidth=2
  Sum1 : Sum  Inputs=++-  SaturateOnIntegerOverflow=on  InputSameDT=on
  edot^2 : Product  Inputs=/**  SaturateOnIntegerOverflow=on  RndMeth=Zero  InputSameDT=on
  Firefct2 : Outport
  wires:
  Sum1/1 -> Firefct2/1
  Select e/1 -> Sum1/2  "e"
  Constant2/1 -> Sum1/1
  1/(2*alph)/1 -> Sum1/3
  e and edot/1 -> Select edot/1, Select e/1
  NofJets/1 -> edot^2/1
  Select edot/1 -> edot^2/3, edot^2/2  "edot"
  edot^2/1 -> 1/(2*alph)/1  "edot^2"

== system aero_dap3dof/Reaction Jet Control/v Control Law/Subsystem3 ==
  note: Coastfct2
      | This function establishes when the jets are to be turned off (coasting)
      | Coastfct1 = e + edot ^2/(2*N*alphs) + DB
  e and edot : Inport  Orientation=down  Port=1  LatchInput=off
  NofJets : Inport  Port=2  LatchInput=off
  1/(2*alph) : Gain  Gain=1/(2*alphs)  SaturateOnIntegerOverflow=on
  Constant2 : Constant  Value=DB
  Select e : Selector  Elements=[1]  InputPortWidth=2
  Select edot : Selector  Elements=[2]  InputPortWidth=2
  Sum1 : Sum  Inputs=+++  SaturateOnIntegerOverflow=on  InputSameDT=on
  edot^2 : Product  Inputs=/**  SaturateOnIntegerOverflow=on  RndMeth=Zero  InputSameDT=on
  Coastfct2 : Outport
  wires:
  Sum1/1 -> Coastfct2/1
  Select e/1 -> Sum1/2  "e"
  Constant2/1 -> Sum1/1
  1/(2*alph)/1 -> Sum1/3
  e and edot/1 -> Select edot/1, Select e/1
  NofJets/1 -> edot^2/1
  Select edot/1 -> edot^2/3, edot^2/2  "edot"
  edot^2/1 -> 1/(2*alph)/1  "edot^2"

== stateflow chart Reaction Jet Control/u Control Law/Chart ==
  settings: updateMethod=DISCRETE  sampleTime=delt
  state Wait_for_stable_rate
  state Start
  state Fire_region_1
    en: jets=-Nofjets;
    ton=tjcalc+tjcalc1;
  state Coast_region_2
    en: jets=0;
    ton=0;
    enable=0;
  state Skip_a_Sample_2
    en:count--;
  state Skip_a_Sample_1
    en:count--;
  state Coast_region_1
    en: jets=0;
    ton=0;
    enable=0;
  state Fire_region_2
    en: jets=Nofjets;
    ton=tjcalc-tjcalc1;
  Wait_for_stable_rate -> Start : [count==0]
  (default) -> Wait_for_stable_rate : /count=2;
  Wait_for_stable_rate -> Wait_for_stable_rate : /count--;
  Start -> Fire_region_2 : [ (e[1]<0 & Firefct2<0) | (e[1]>0 & Coastfct2>0) ]
  Start -> Coast_region_1 : [ (e[1]<0 & Coastfct1<=0 & Firefct2>0) ]
  Start -> Coast_region_2 : [ (e[1]>0 & Coastfct2>=0 & Firefct1<0) ]
  Start -> Fire_region_1 : [ (e[1]>0 & Firefct1>0) | (e[1]<0 & Coastfct1<0) ]
  Coast_region_2 -> Fire_region_1 : [e[1]>0 & Firefct1>0]
  Skip_a_Sample_2 -> Coast_region_2 : [count==0]
  Fire_region_1 -> Fire_region_1
  Fire_region_1 -> (junction 11) : [ton<2*delt]{enable=1;}
  Fire_region_1 -> Coast_region_1 : [e[1]<0 & Coastfct1<=0]
  (junction 12) -> Coast_region_2 : {enable=0;}
  Fire_region_2 -> Coast_region_2 : [e[1]>0 & Coastfct2>0]
  (junction 11) -> Coast_region_1 : {enable=0;}
  Skip_a_Sample_2 -> Skip_a_Sample_2 : /ton=ton-delt;
  (junction 11) -> Skip_a_Sample_1 : [ton>tmin]{count=2;}
  (junction 12) -> Skip_a_Sample_2 : [ton>tmin]{count=2;}
  Skip_a_Sample_1 -> Skip_a_Sample_1 : /ton=ton-delt;
  Skip_a_Sample_1 -> Coast_region_1 : [count==0]
  Fire_region_2 -> (junction 12) : [ton<2*delt]{enable=1;}
  Coast_region_1 -> Fire_region_2 : [e[1]<0 & Firefct2<0]
  Fire_region_2 -> Fire_region_2
  data: jets output double size=1; Nofjets input double size=1; e input double size=2; enable output double size=1; ton output double size=1; Firefct1 input double size=1; Coastfct1 input double size=1; Firefct2 input double size=1; Coastfct2 input double size=1; tjcalc1 input double size=1; tjcalc input double size=1; tmin parameter double size=1; delt parameter double size=1; count local double size=1

== stateflow chart Reaction Jet Control/v Control Law/Chart ==
  settings: updateMethod=DISCRETE  sampleTime=delt
  state Wait_for_stable_rate
  state Start
  state Fire_region_1
    en: jets=-Nofjets;
    ton=tjcalc+tjcalc1;
  state Coast_region_2
    en: jets=0;
    ton=0;
    enable=0;
  state Skip_a_Sample_2
    en:count--;
  state Skip_a_Sample_1
    en:count--;
  state Coast_region_1
    en: jets=0;
    ton=0;
    enable=0;
  state Fire_region_2
    en: jets=Nofjets;
    ton=tjcalc-tjcalc1;
  Wait_for_stable_rate -> Start : [count==0]
  (default) -> Wait_for_stable_rate : /count=2;
  Wait_for_stable_rate -> Wait_for_stable_rate : /count--;
  Start -> Fire_region_2 : [ (e[1]<0 & Firefct2<0) | (e[1]>0 & Coastfct2>0) ]
  Start -> Coast_region_1 : [ (e[1]<0 & Coastfct1<=0 & Firefct2>0) ]
  Start -> Coast_region_2 : [ (e[1]>0 & Coastfct2>=0 & Firefct1<0) ]
  Start -> Fire_region_1 : [ (e[1]>0 & Firefct1>0) | (e[1]<0 & Coastfct1<0) ]
  Coast_region_2 -> Fire_region_1 : [e[1]>0 & Firefct1>0]
  Skip_a_Sample_2 -> Coast_region_2 : [count==0]
  Fire_region_1 -> Fire_region_1
  Fire_region_1 -> (junction 60) : [ton<2*delt]{enable=1;}
  Fire_region_1 -> Coast_region_1 : [e[1]<0 & Coastfct1<=0]
  (junction 61) -> Coast_region_2 : {enable=0;}
  Fire_region_2 -> Coast_region_2 : [e[1]>0 & Coastfct2>0]
  (junction 60) -> Coast_region_1 : {enable=0;}
  Skip_a_Sample_2 -> Skip_a_Sample_2 : /ton=ton-delt;
  (junction 60) -> Skip_a_Sample_1 : [ton>tmin]{count=2;}
  (junction 61) -> Skip_a_Sample_2 : [ton>tmin]{count=2;}
  Skip_a_Sample_1 -> Skip_a_Sample_1 : /ton=ton-delt;
  Skip_a_Sample_1 -> Coast_region_1 : [count==0]
  Fire_region_2 -> (junction 61) : [ton<2*delt]{enable=1;}
  Coast_region_1 -> Fire_region_2 : [e[1]<0 & Firefct2<0]
  Fire_region_2 -> Fire_region_2
  data: jets output double size=1; Nofjets input double size=1; e input double size=2; enable output double size=1; ton output double size=1; Firefct1 input double size=1; Coastfct1 input double size=1; Firefct2 input double size=1; Coastfct2 input double size=1; tjcalc1 input double size=1; tjcalc input double size=1; tmin parameter double size=1; delt parameter double size=1; count local double size=1

== stateflow chart Reaction Jet Control/Yaw Control Law/Chart ==
  settings: updateMethod=DISCRETE  sampleTime=delt
  state Wait_for_stable_rate
  state Start
  state Fire_region_1
    en: jets=-Nofjets;
    ton=tjcalc+tjcalc1;
  state Coast_region_2
    en: jets=0;
    ton=0;
    enable=0;
  state Skip_a_Sample_2
    en:count--;
  state Skip_a_Sample_1
    en:count--;
  state Coast_region_1
    en: jets=0;
    ton=0;
    enable=0;
  state Fire_region_2
    en: jets=Nofjets;
    ton=tjcalc-tjcalc1;
  Wait_for_stable_rate -> Start : [count==0]
  (default) -> Wait_for_stable_rate : /count=2;
  Wait_for_stable_rate -> Wait_for_stable_rate : /count--;
  Start -> Fire_region_2 : [ (e[1]<0 & Firefct2<0) | (e[1]>0 & Coastfct2>0) ]
  Start -> Coast_region_1 : [ (e[1]<0 & Coastfct1<=0 & Firefct2>0) ]
  Start -> Coast_region_2 : [ (e[1]>0 & Coastfct2>=0 & Firefct1<0) ]
  Start -> Fire_region_1 : [ (e[1]>0 & Firefct1>0) | (e[1]<0 & Coastfct1<0) ]
  Coast_region_2 -> Fire_region_1 : [e[1]>0 & Firefct1>0]
  Skip_a_Sample_2 -> Coast_region_2 : [count==0]
  Fire_region_1 -> Fire_region_1
  Fire_region_1 -> (junction 109) : [ton<2*delt]{enable=1;}
  Fire_region_1 -> Coast_region_1 : [e[1]<0 & Coastfct1<=0]
  (junction 110) -> Coast_region_2 : {enable=0;}
  Fire_region_2 -> Coast_region_2 : [e[1]>0 & Coastfct2>0]
  (junction 109) -> Coast_region_1 : {enable=0;}
  Skip_a_Sample_2 -> Skip_a_Sample_2 : /ton=ton-delt;
  (junction 109) -> Skip_a_Sample_1 : [ton>tmin]{count=2;}
  (junction 110) -> Skip_a_Sample_2 : [ton>tmin]{count=2;}
  Skip_a_Sample_1 -> Skip_a_Sample_1 : /ton=ton-delt;
  Skip_a_Sample_1 -> Coast_region_1 : [count==0]
  Fire_region_2 -> (junction 110) : [ton<2*delt]{enable=1;}
  Coast_region_1 -> Fire_region_2 : [e[1]<0 & Firefct2<0]
  Fire_region_2 -> Fire_region_2
  data: jets output double size=1; Nofjets input double size=1; e input double size=2; enable output double size=1; ton output double size=1; Firefct1 input double size=1; Coastfct1 input double size=1; Firefct2 input double size=1; Coastfct2 input double size=1; tjcalc1 input double size=1; tjcalc input double size=1; tmin parameter double size=1; delt parameter double size=1; count local double size=1
